simulink model "robot_reglage_couple_conecyl"  (R2017a)
settings: Solver=VariableStepAuto  StartTime=0.0  StopTime=500  RelTol=1e-3
values from neighbouring files (symbols this model uses):
  F1 = 60    [robot.m]
  F2 = 60    [robot.m]
  F3 = 15    [robot.m]
  I233 = 2    [robot.m]
  I333 = 0.2    [robot.m]
  k1 = 100    [robot.m]
  k2 = 100    [robot.m]
  k3 = 10    [robot.m]
  Kd = 4    [robot.m]
  Kd2 = 3    [robot.m]
  Kd3 = 3    [robot.m]
  Kp = 2    [robot.m]
  Kp2 = 2    [robot.m]
  Kp3 = 3    [robot.m]
  l00 = 0.2    [robot.m]
  L1 = 0.5    [robot.m]
  L2 = 1    [robot.m]
  l22 = 0.5    [robot.m]
  l33 = 0.5    [robot.m]
  m1 = 10    [robot.m]
  m2 = 5    [robot.m]
  m3 = 5    [robot.m]
  P = 4    [robot.m]
  R = 0.5    [robot.m]
  w = 0.1    [robot.m]
  x0 = 1    [robot.m]
  y0 = L2    (= 1)    [robot.m]
  z0 = L1    (= 0.5)    [robot.m]
settings Model: Creator=massona  LastModifiedBy=massona
settings DataIOCC: Refine=100

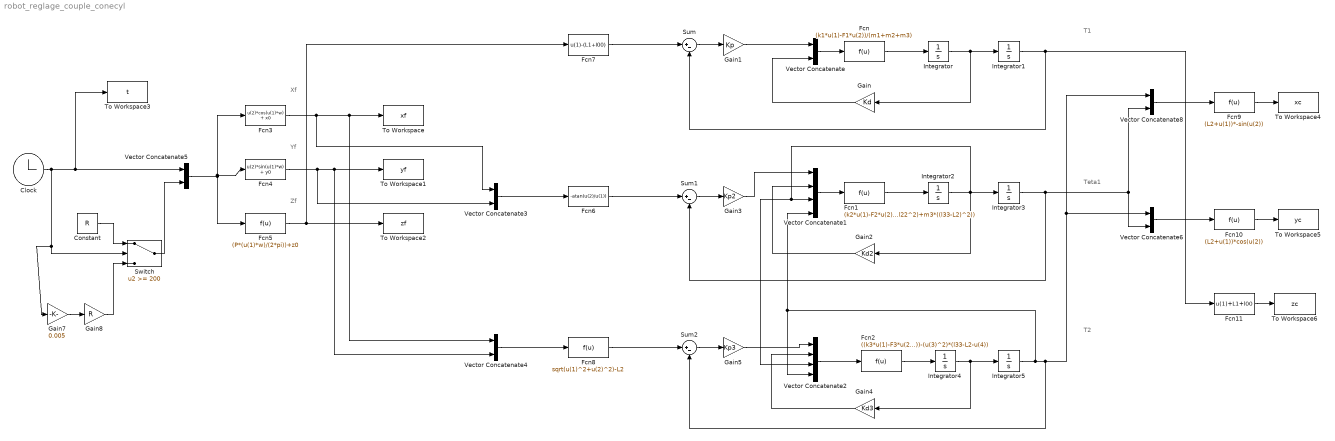
== system robot_reglage_couple_conecyl ==
  note: T1
  note: Teta1
  note: T2
  note: Zf
  note: Xf
  note: Yf
  Clock : Clock
  Constant : Constant  Value=R
  Fcn : Fcn  Expr=(k1*u(1)-F1*u(2))/(m1+m2+m3)
  Fcn1 : Fcn  Expr=(k2*u(1)-F2*u(2)+2*m3*(l33-u(4)-L2)*u(3)*u(4))/(I233+I333+m2*(l22^2)+m3*((l33-L2)^2))
  Fcn10 : Fcn  Expr=(L2+u(1))*cos(u(2))
  Fcn11 : Fcn  Expr=u(1)+L1+l00
  Fcn2 : Fcn  Expr=((k3*u(1)-F3*u(2))/(m3))-(u(3)^2)*(l33-L2-u(4))
  Fcn3 : Fcn  Expr=u(2)*cos(u(1)*w) + x0
  Fcn4 : Fcn  Expr=u(2)*sin(u(1)*w) + y0
  Fcn5 : Fcn  Expr=(P*(u(1)*w)/(2*pi))+z0
  Fcn6 : Fcn  Expr=-atan(u(2)/u(1))
  Fcn7 : Fcn  Expr=u(1)-(L1+l00)
  Fcn8 : Fcn  Expr=sqrt(u(1)^2+u(2)^2)-L2
  Fcn9 : Fcn  Expr=(L2+u(1))*-sin(u(2))
  Gain : Gain  Gain=Kd
  Gain1 : Gain  Gain=Kp
  Gain2 : Gain  Gain=Kd2
  Gain3 : Gain  Gain=Kp2
  Gain4 : Gain  Gain=Kd3
  Gain5 : Gain  Gain=Kp3
  Gain7 : Gain  Gain=0.005
  Gain8 : Gain  Gain=R
  Integrator{,1..5} (6 alike) : Integrator
  Sum : Sum  Inputs=|+-
  Sum1 : Sum  Inputs=|+-
  Sum2 : Sum  Inputs=|+-
  Switch : Switch  Threshold=200
  To Workspace : ToWorkspace  VariableName=xf  SampleTime=-1
  To Workspace1 : ToWorkspace  VariableName=yf  SampleTime=-1
  To Workspace2 : ToWorkspace  VariableName=zf  SampleTime=-1
  To Workspace3 : ToWorkspace  VariableName=t  SampleTime=-1
  To Workspace4 : ToWorkspace  VariableName=xc  SampleTime=-1
  To Workspace5 : ToWorkspace  VariableName=yc  SampleTime=-1
  To Workspace6 : ToWorkspace  VariableName=zc  SampleTime=-1
  Vector Concatenate{,3..6,8} (6 alike) : Concatenate
  Vector Concatenate1 : Concatenate  NumInputs=4
  Vector Concatenate2 : Concatenate  NumInputs=4
  wires:
  Vector Concatenate/1 -> Fcn/1
  Fcn/1 -> Integrator/1
  Integrator/1 -> Integrator1/1, Gain/1
  Gain/1 -> Vector Concatenate/2
  Gain1/1 -> Vector Concatenate/1
  Sum/1 -> Gain1/1
  Integrator1/1 -> Fcn11/1, Sum/2
  Fcn3/1 -> Vector Concatenate3/1, Vector Concatenate4/1, To Workspace/1
  Fcn4/1 -> Vector Concatenate3/2, Vector Concatenate4/2, To Workspace1/1
  Integrator3/1 -> Sum1/2, Vector Concatenate6/2, Vector Concatenate8/2
  Sum1/1 -> Gain3/1
  Gain3/1 -> Vector Concatenate1/1
  Gain2/1 -> Vector Concatenate1/2
  Fcn1/1 -> Integrator2/1
  Vector Concatenate1/1 -> Fcn1/1
  Vector Concatenate2/1 -> Fcn2/1
  Fcn2/1 -> Integrator4/1
  Integrator4/1 -> Integrator5/1, Gain4/1
  Gain4/1 -> Vector Concatenate2/2
  Gain5/1 -> Vector Concatenate2/1
  Sum2/1 -> Gain5/1
  Fcn5/1 -> To Workspace2/1, Fcn7/1
  Fcn6/1 -> Sum1/1
  Vector Concatenate3/1 -> Fcn6/1
  Fcn7/1 -> Sum/1
  Vector Concatenate4/1 -> Fcn8/1
  Fcn8/1 -> Sum2/1
  Fcn9/1 -> To Workspace4/1
  Fcn10/1 -> To Workspace5/1
  Fcn11/1 -> To Workspace6/1
  Vector Concatenate8/1 -> Fcn9/1
  Integrator5/1 -> Vector Concatenate2/4, Vector Concatenate1/4, Sum2/2, Vector Concatenate6/1, Vector Concatenate8/1
  Vector Concatenate6/1 -> Fcn10/1
  Integrator2/1 -> Gain2/1, Integrator3/1, Vector Concatenate2/3, Vector Concatenate1/3
  Clock/1 -> Gain7/1, Switch/2, Vector Concatenate5/1, To Workspace3/1
  Gain7/1 -> Gain8/1
  Gain8/1 -> Switch/3
  Vector Concatenate5/1 -> Fcn5/1, Fcn4/1, Fcn3/1
  Constant/1 -> Switch/1
  Switch/1 -> Vector Concatenate5/2
